simulink model "model_task_2_7"  (Simulink 8.5)
settings: Solver=ode45  StartTime=tstart  StopTime=tstop  RelTol=1e-3
values from neighbouring files (symbols this model uses):
  c = 1    [run_task_2_7.m]
  c_m = 5467    [run_task_2_7.m]
  c_u = -0.0018    [run_task_2_7.m]
  c_uu = 1.0378    [run_task_2_7.m]
  K = -0.0590    (= -0.059)    [run_task_2_7.m]
  K_d_c = 3*lambda_c    (= 0.3)    [run_task_2_7.m]
  k_i = lambda^2    [run_task_2_7.m]
  K_i_c = lambda_c^3    (= 0.001)    [run_task_2_7.m]
  k_p = 2*lambda    [run_task_2_7.m]
  K_p_c = 3*lambda_c^2    (= 0.03)    [run_task_2_7.m]
  omega = 0.01    [run_task_2_7.m]
  omega_c = 0.1    [run_task_2_7.m]
  psi0 = 150*deg2rad    (= 2.61799387799)    [run_task_2_7.m]
  r0 = 0    [run_task_2_7.m]
  T = 111.5778    [run_task_2_7.m]
  tsamp = 10    [run_task_2_7.m]
  v0 = [6.63 0]'    [run_task_2_7.m]
  zeta = 1    [run_task_2_7.m]
  zeta_c = 1    [run_task_2_7.m]
undefined symbols (not defined in the file or in its folder): guidance_control, msfartoystyring
undefined symbols (not defined in the file): p0
settings Model: Creator=christh  LastModifiedBy=torsteik  CovSFcnEnable=off  ExtModeAutoUpdateStatusClock=off
settings DataIOCC: SignalLoggingSaveFormat=Dataset
settings OptimizationCC: InitFltsAndDblsToZero=on
settings DebuggingCC: SolverPrmCheckMsg=warning  FcnCallInpInsideContextMsg=UseLocalSettings
settings ConfigComp: CovMetricSettings=dw  CovHtmlReporting=on  CovSaveCumulativeToWorkspaceVar=on  CovSaveSingleToWorkspaceVar=on  CovModelRefEnable=Off  CovExternalEMLEnable=off

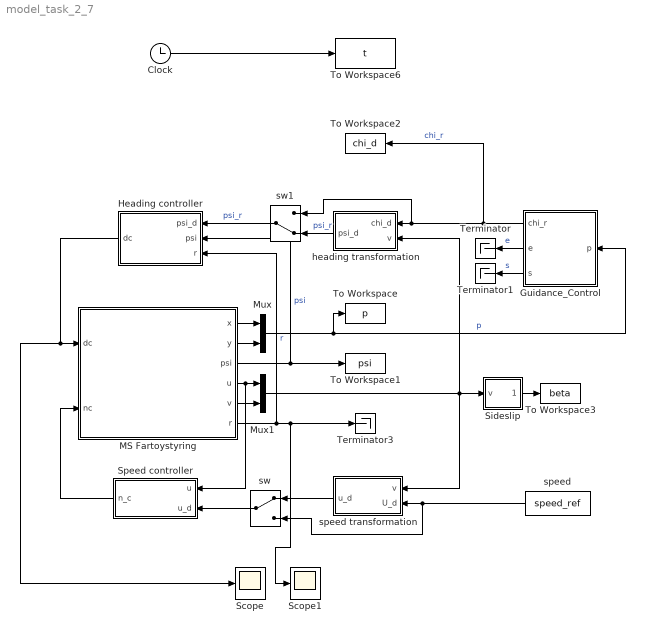
== system model_task_2_7 ==
  Clock : Clock
  Guidance_Control : Subsystem
  Heading controller : Subsystem
  MS Fartoystyring : Subsystem  mask(MS Fartoystyring for Assignment 3 G&C){x0=p0(1), y0=p0(2), u0=v0(1), v0=v0(2), psi0=psi0, r0=r0, c=c}
      mask prompts: x0 "x(t0) (m)"; y0 "y(t0) (m)"; u0 "u(t0) (m/s)"; v0 "v(t0) (m/s)"; psi0 "psi(t0) (rad)"; r0 "r(t0) (rad/s)"; c "current (0 or 1)"
      mask help:
      | Block corresponding to Figure 1 in the assignment text. Gives the response of the ship.
      |
      | The design speed of MS Fartoystyring is u=8.23 m/s.
      |
      | Input:
      | dc: commanded rudder (rad), dmax=25*pi/180
      | nc: commanded shaft speed (rad/s), nmax=85*2*pi/60
      |
      | Output:
      | x: north pos (m)
      | y: east pos (m)
      | u: surge (m/s)
      | v: sway (m/s)
      | psi: heading (rad)
      | r: yaw (rad/s)
      mask Help: Comments, bugs and help requests can be directed to the TA. Email on course website.
  Mux : Mux  Inputs=2
  Mux1 : Mux  Inputs=2
  Scope : Scope
  Scope1 : Scope
  Sideslip : Subsystem
  Speed controller : Subsystem
  Terminator : Terminator
  Terminator1 : Terminator
  Terminator3 : Terminator
  To Workspace : ToWorkspace  VariableName=p  SampleTime=tsamp
  To Workspace1 : ToWorkspace  VariableName=psi  SampleTime=tsamp
  To Workspace2 : ToWorkspace  VariableName=chi_d  SampleTime=tsamp
  To Workspace3 : ToWorkspace  VariableName=beta  SampleTime=tsamp
  To Workspace6 : ToWorkspace  VariableName=t  SampleTime=tsamp
  heading transformation : Subsystem
  speed : FromWorkspace  VariableName=speed_ref  SampleTime=0
  speed transformation : Subsystem
  sw : ManualSwitch
  sw1 : ManualSwitch  CurrentSetting=0
  wires:
  Clock/1 -> To Workspace6/1
  MS Fartoystyring/1(x) -> Mux/1
  MS Fartoystyring/2(y) -> Mux/2
  MS Fartoystyring/4(u) -> Speed controller/1(u), Mux1/1
  MS Fartoystyring/5(v) -> Mux1/2
  Mux/1 -> To Workspace/1, Guidance_Control/1(p)  "p"
  MS Fartoystyring/3(psi) -> To Workspace1/1, Heading controller/2(psi)  "psi"
  MS Fartoystyring/6(r) -> Scope1/1, Terminator3/1, Heading controller/3(r)  "r"
  Speed controller/1(n_c) -> MS Fartoystyring/2(nc)
  Heading controller/1(dc) -> Scope/1, MS Fartoystyring/1(dc)
  Guidance_Control/1(chi_r) -> To Workspace2/1, sw1/1, heading transformation/1(chi_d)  "chi_r"
  Guidance_Control/2(e) -> Terminator/1  "e"
  Guidance_Control/3(s) -> Terminator1/1  "s"
  sw1/1 -> Heading controller/1(psi_d)  "psi_r"
  Mux1/1 -> speed transformation/1(v), Sideslip/1(v), heading transformation/2(v)
  Sideslip/1(beta) -> To Workspace3/1
  speed/1 -> sw/2, speed transformation/2(U_d)
  sw/1 -> Speed controller/2(u_d)
  speed transformation/1(u_d) -> sw/1
  heading transformation/1(psi_d) -> sw1/2  "psi_r"

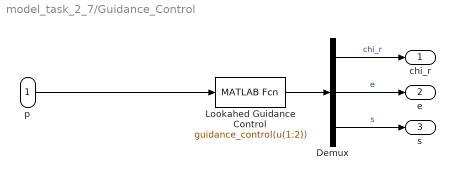
== system model_task_2_7/Guidance_Control ==
  p : Inport
  Demux : Demux  Outputs=3
  Lookahed Guidance Control : MATLABFcn  MATLABFcn=guidance_control(u(1:2))  OutputDimensions=3
  chi_r : Outport
  e : Outport  Port=2
  s : Outport  Port=3
  wires:
  Lookahed Guidance Control/1 -> Demux/1
  Demux/2 -> e/1  "e"
  Demux/1 -> chi_r/1  "chi_r"
  Demux/3 -> s/1  "s"
  p/1 -> Lookahed Guidance Control/1

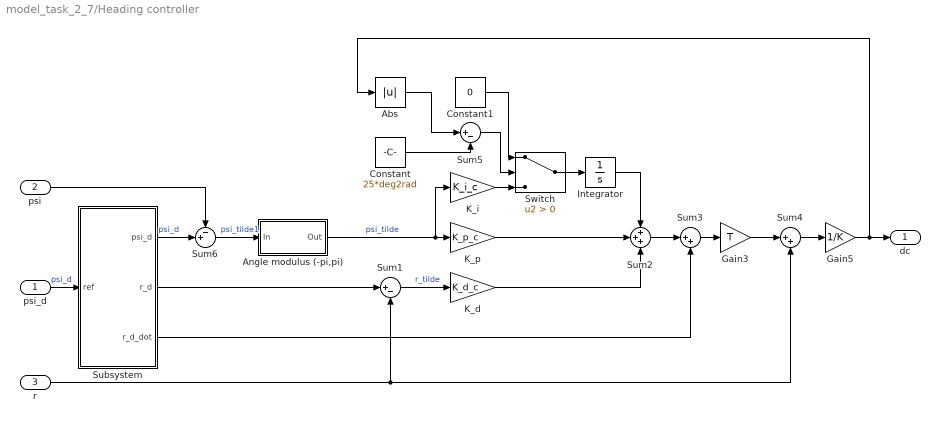
== system model_task_2_7/Heading controller ==
  psi_d : Inport
  psi : Inport  Port=2
  r : Inport  Port=3
  Abs : Abs
  Angle modulus (-pi,pi) : Subsystem
  Constant : Constant  Value=25*deg2rad
  Constant1 : Constant  Value=0
  Gain3 : Gain  Gain=T
  Gain5 : Gain  Gain=1/K
  Integrator : Integrator  LimitOutput=on  UpperSaturationLimit=deg2rad*25*abs(K)/T  LowerSaturationLimit=-deg2rad*25*abs(K)/T
  K_d : Gain  Gain=K_d_c
  K_i : Gain  Gain=K_i_c
  K_p : Gain  Gain=K_p_c
  Subsystem : Subsystem
  Sum1 : Sum  Inputs=|+-
  Sum2 : Sum  Inputs=+++
  Sum3 : Sum  Inputs=|++
  Sum4 : Sum  Inputs=|++
  Sum5 : Sum  Inputs=|+-
  Sum6 : Sum  Inputs=-+|
  Switch : Switch  Criteria=u2 > Threshold
  dc : Outport
  wires:
  Sum1/1 -> K_d/1  "r_tilde"
  Angle modulus (-pi,pi)/1(Out) -> K_i/1, K_p/1  "psi_tilde"
  Subsystem/2(r_d) -> Sum1/1
  K_p/1 -> Sum2/2
  Sum2/1 -> Sum3/1
  K_d/1 -> Sum2/3
  Subsystem/3(r_d_dot) -> Sum3/2
  Sum3/1 -> Gain3/1
  Gain3/1 -> Sum4/1
  r/1 -> Sum4/2, Sum1/2
  Gain5/1 -> Abs/1, dc/1
  Sum4/1 -> Gain5/1
  Integrator/1 -> Sum2/1
  Abs/1 -> Sum5/1
  Sum5/1 -> Switch/2
  Constant/1 -> Sum5/2
  Constant1/1 -> Switch/1
  K_i/1 -> Switch/3
  Switch/1 -> Integrator/1
  psi_d/1 -> Subsystem/1(ref)  "psi_d"
  Sum6/1 -> Angle modulus (-pi,pi)/1(In)  "psi_tilde1"
  psi/1 -> Sum6/1
  Subsystem/1(psi_d) -> Sum6/2  "psi_d"

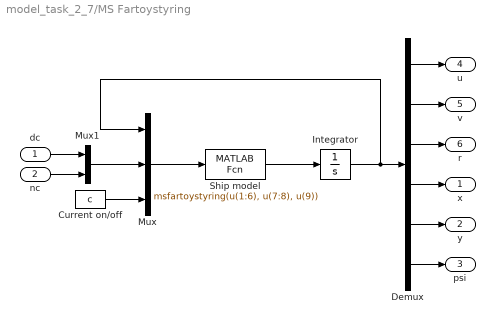
== system model_task_2_7/MS Fartoystyring ==
  dc : Inport
  nc : Inport  Port=2
  Current on/off : Constant  Value=c
  Demux : Demux  Outputs=6
  Integrator : Integrator  InitialCondition=[u0 v0 r0 x0 y0 psi0]'
  Mux : Mux  Inputs=3
  Mux1 : Mux  Inputs=2
  Ship model : MATLABFcn  MATLABFcn=msfartoystyring(u(1:6), u(7:8), u(9))  OutputDimensions=6
  x : Outport
  y : Outport  Port=2
  psi : Outport  Port=3
  u : Outport  Port=4
  v : Outport  Port=5
  r : Outport  Port=6
  wires:
  Integrator/1 -> Mux/1, Demux/1
  Mux1/1 -> Mux/2
  dc/1 -> Mux1/1
  nc/1 -> Mux1/2
  Demux/1 -> u/1
  Demux/2 -> v/1
  Demux/3 -> r/1
  Demux/4 -> x/1
  Demux/5 -> y/1
  Demux/6 -> psi/1
  Current on/off/1 -> Mux/3
  Ship model/1 -> Integrator/1
  Mux/1 -> Ship model/1

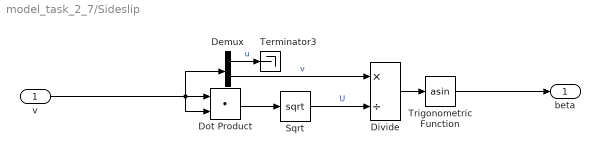
== system model_task_2_7/Sideslip ==
  v : Inport
  Demux : Demux  Outputs=2
  Divide : Product  Inputs=*/
  Dot Product : DotProduct  InputSameDT=on  OutDataTypeStr=Inherit: Inherit via internal rule
  Sqrt : Sqrt  SaturateOnIntegerOverflow=on
  Terminator3 : Terminator
  Trigonometric Function : Trigonometry  Operator=asin
  beta : Outport
  wires:
  v/1 -> Dot Product/2, Demux/1, Dot Product/1
  Demux/2 -> Divide/1  "v"
  Sqrt/1 -> Divide/2  "U"
  Trigonometric Function/1 -> beta/1
  Dot Product/1 -> Sqrt/1
  Divide/1 -> Trigonometric Function/1
  Demux/1 -> Terminator3/1  "u"

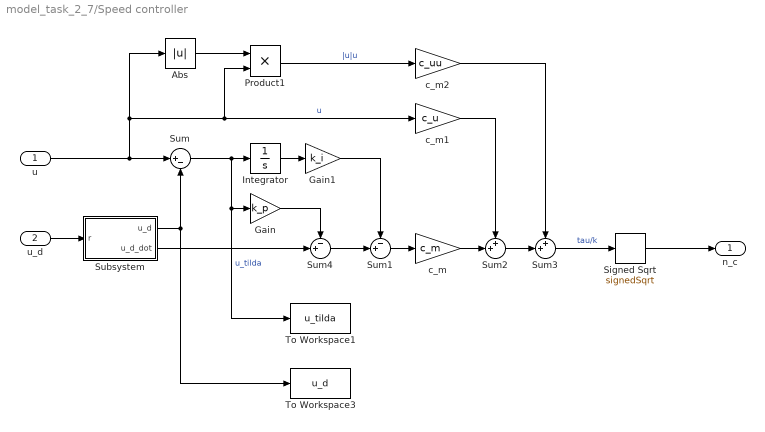
== system model_task_2_7/Speed controller ==
  u : Inport
  u_d : Inport  Port=2
  Abs : Abs
  Gain : Gain  Gain=k_p
  Gain1 : Gain  Gain=k_i
  Integrator : Integrator
  Product1 : Product
  Signed Sqrt : Sqrt  Operator=signedSqrt  SaturateOnIntegerOverflow=on
  Subsystem : Subsystem
  Sum : Sum  Inputs=|+-
  Sum1 : Sum  Inputs=-+|
  Sum2 : Sum  Inputs=++|
  Sum3 : Sum  Inputs=++|
  Sum4 : Sum  Inputs=-+|
  To Workspace1 : ToWorkspace  VariableName=u_tilda  SampleTime=tsamp
  To Workspace3 : ToWorkspace  VariableName=u_d  SampleTime=tsamp
  c_m : Gain  Gain=c_m
  c_m1 : Gain  Gain=c_u
  c_m2 : Gain  Gain=c_uu
  n_c : Outport
  wires:
  u_d/1 -> Subsystem/1(r)
  u/1 -> Sum/1, Abs/1, Product1/2, c_m1/1  "u"
  Subsystem/1(u_d) -> Sum/2, To Workspace3/1
  Sum/1 -> Gain/1, To Workspace1/1, Integrator/1  "u_tilda"
  Subsystem/2(u_d_dot) -> Sum4/2
  Integrator/1 -> Gain1/1
  Sum1/1 -> c_m/1
  c_m/1 -> Sum2/2
  c_m1/1 -> Sum2/1
  Sum2/1 -> Sum3/2
  c_m2/1 -> Sum3/1
  Abs/1 -> Product1/1
  Product1/1 -> c_m2/1  "|u|u"
  Sum3/1 -> Signed Sqrt/1  "tau/k"
  Signed Sqrt/1 -> n_c/1
  Sum4/1 -> Sum1/2
  Gain1/1 -> Sum1/1
  Gain/1 -> Sum4/1

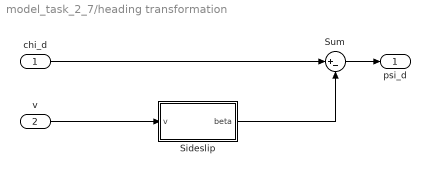
== system model_task_2_7/heading transformation ==
  chi_d : Inport
  v : Inport  Port=2
  Sideslip : Subsystem
  Sum : Sum  Inputs=|+-
  psi_d : Outport
  wires:
  chi_d/1 -> Sum/1
  v/1 -> Sideslip/1(v)
  Sum/1 -> psi_d/1
  Sideslip/1(beta) -> Sum/2

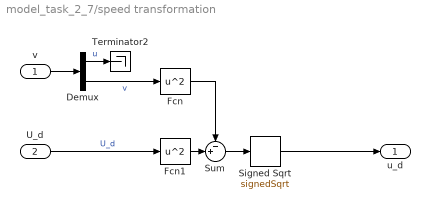
== system model_task_2_7/speed transformation ==
  v : Inport
  U_d : Inport  Port=2
  Demux : Demux  Outputs=2
  Fcn : Fcn  Expr=u^2
  Fcn1 : Fcn  Expr=u^2
  Signed Sqrt : Sqrt  Operator=signedSqrt  SaturateOnIntegerOverflow=on
  Sum : Sum  Inputs=-+|
  Terminator2 : Terminator
  u_d : Outport
  wires:
  Demux/1 -> Terminator2/1  "u"
  v/1 -> Demux/1
  Fcn/1 -> Sum/1
  Demux/2 -> Fcn/1  "v"
  Fcn1/1 -> Sum/2
  U_d/1 -> Fcn1/1  "U_d"
  Sum/1 -> Signed Sqrt/1
  Signed Sqrt/1 -> u_d/1

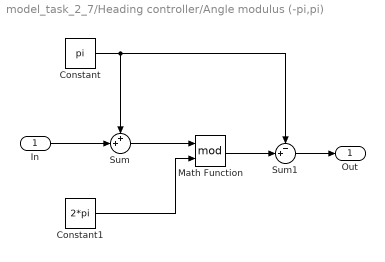
== system model_task_2_7/Heading controller/Angle modulus (-pi,pi) ==
  In : Inport
  Constant : Constant  Value=pi
  Constant1 : Constant  Value=2*pi
  Math Function : Math  Operator=mod  SaturateOnIntegerOverflow=on
  Sum : Sum  Inputs=++|
  Sum1 : Sum  Inputs=-+|
  Out : Outport
  wires:
  Math Function/1 -> Sum1/2
  Sum/1 -> Math Function/1
  Constant/1 -> Sum1/1, Sum/1
  In/1 -> Sum/2
  Sum1/1 -> Out/1
  Constant1/1 -> Math Function/2

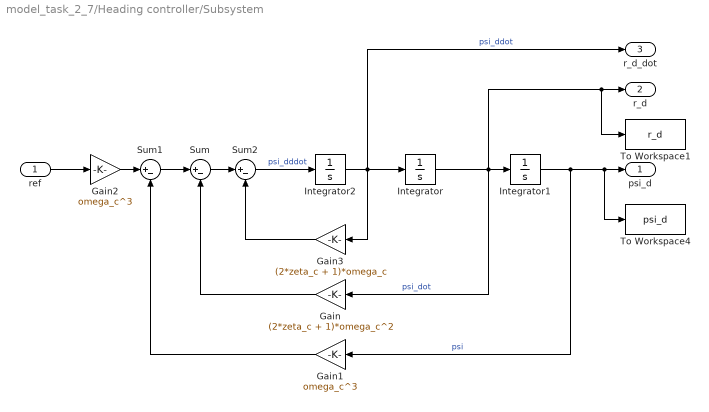
== system model_task_2_7/Heading controller/Subsystem ==
  ref : Inport
  Gain : Gain  Gain=(2*zeta_c + 1)*omega_c^2
  Gain1 : Gain  Gain=omega_c^3
  Gain2 : Gain  Gain=omega_c^3
  Gain3 : Gain  Gain=(2*zeta_c + 1)*omega_c
  Integrator : Integrator
  Integrator1 : Integrator  InitialCondition=psi0
  Integrator2 : Integrator
  Sum : Sum  Inputs=|+-
  Sum1 : Sum  Inputs=|+-
  Sum2 : Sum  Inputs=|+-
  To Workspace1 : ToWorkspace  VariableName=r_d  SampleTime=tsamp
  To Workspace4 : ToWorkspace  VariableName=psi_d  SampleTime=tsamp
  psi_d : Outport
  r_d : Outport  Port=2
  r_d_dot : Outport  Port=3
  wires:
  Integrator1/1 -> psi_d/1, To Workspace4/1, Gain1/1  "psi"
  Sum1/1 -> Sum/1
  Integrator2/1 -> Gain3/1, r_d_dot/1, Integrator/1  "psi_ddot"
  Gain1/1 -> Sum1/2
  ref/1 -> Gain2/1
  Gain/1 -> Sum/2
  Integrator/1 -> To Workspace1/1, r_d/1, Gain/1, Integrator1/1  "psi_dot"
  Gain2/1 -> Sum1/1
  Sum2/1 -> Integrator2/1  "psi_dddot"
  Sum/1 -> Sum2/1
  Gain3/1 -> Sum2/2

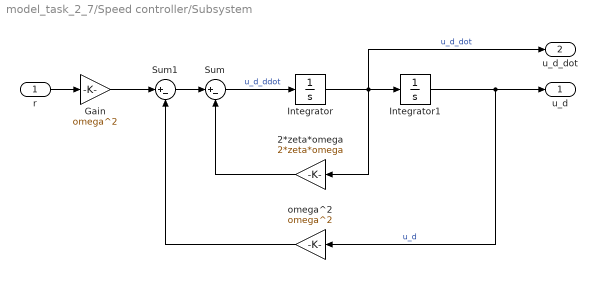
== system model_task_2_7/Speed controller/Subsystem ==
  r : Inport
  2*zeta*omega : Gain  Gain=2*zeta*omega
  Gain : Gain  Gain=omega^2
  Integrator : Integrator
  Integrator1 : Integrator  InitialCondition=v0(1)
  Sum : Sum  Inputs=|+-
  Sum1 : Sum  Inputs=|+-
  omega^2 : Gain  Gain=omega^2
  u_d : Outport
  u_d_dot : Outport  Port=2
  wires:
  Integrator/1 -> u_d_dot/1, Integrator1/1, 2*zeta*omega/1  "u_d_dot"
  Integrator1/1 -> u_d/1, omega^2/1  "u_d"
  Sum/1 -> Integrator/1  "u_d_ddot"
  Sum1/1 -> Sum/1
  2*zeta*omega/1 -> Sum/2
  omega^2/1 -> Sum1/2
  r/1 -> Gain/1
  Gain/1 -> Sum1/1

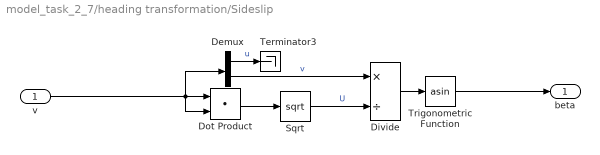
== system model_task_2_7/heading transformation/Sideslip ==
  v : Inport
  Demux : Demux  Outputs=2
  Divide : Product  Inputs=*/
  Dot Product : DotProduct  InputSameDT=on  OutDataTypeStr=Inherit: Inherit via internal rule
  Sqrt : Sqrt  SaturateOnIntegerOverflow=on
  Terminator3 : Terminator
  Trigonometric Function : Trigonometry  Operator=asin
  beta : Outport
  wires:
  v/1 -> Dot Product/2, Demux/1, Dot Product/1
  Demux/2 -> Divide/1  "v"
  Sqrt/1 -> Divide/2  "U"
  Trigonometric Function/1 -> beta/1
  Dot Product/1 -> Sqrt/1
  Divide/1 -> Trigonometric Function/1
  Demux/1 -> Terminator3/1  "u"
